simulink model "MotorSlider"  (R2022b)
settings: Solver=VariableStepAuto  StartTime=0.0  StopTime=10  RelTol=1e-3
InitFcn:
  | init_slider
StopFcn:
  | plot_slider_pos
libraries: fl_lib x13, nesl_utility x6, simulink x2, ee_lib x1
settings Model: Creator=lin-t  LastModifiedBy=ddem325
settings DebuggingCC: UnconnectedInputMsg=warning  UnconnectedOutputMsg=warning  UnconnectedLineMsg=warning
settings ModelReferenceCC: EnableRefExpFcnMdlSchedulingChecks=on
settings RTWCC: DLArmComputeVersion=19.05

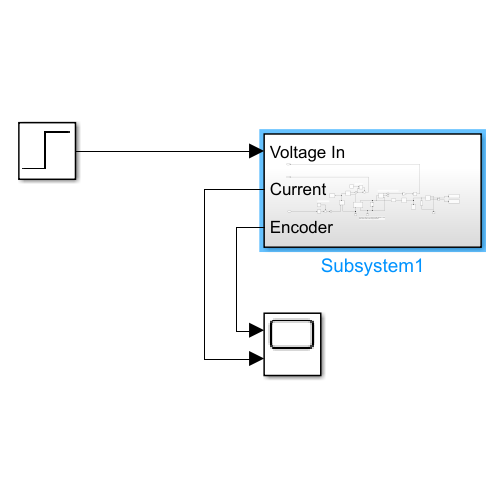
[thumbnail: Simulink's stored preview of the top-level diagram]
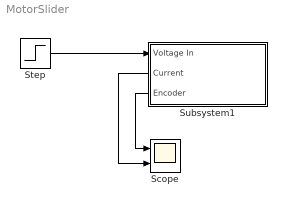
== system MotorSlider ==
  Scope : Scope  NumInputPorts=2
  Step : Step  SampleTime=0
  Subsystem1 : Subsystem
      settings: PortSchema="{\"entries\":[{\"content\":{\"sides\":[{\"content\":{\"connectorIds\":[\"In1\",\"Out1\",\"Out2\"]},\"type\":\"ConnectorPlacement.EquallySpacedRectSide\",\"uuid\":\"37b6e8a3-fab1-42a2-a82e-05d59ddeab9c\"},{\"content\":{\"connectorIds\":[],\"side\":\"RIGHT\"},\"type\":\"ConnectorPlacement.EquallySpacedRectSide\",\"uuid\":\"1ba3cb90-8de0-445d-86e1-8f55e0434744\"},{\"content\":{\"connectorIds\":[],\"side\":\"TOP\"},\"type\":\"ConnectorPlacement.EquallySpacedRectSide\",\"uuid\":\"a1626594-3f4c-461f-b31a-4794292535e7\"}]},\"type\":\"ConnectorPlacement.EquallySpacedConnector\",\"uuid\":\"a2f806fd-1b7f-4e1d-b761-307198229793\"}],\"packageUris\":[\"http://schema.mathworks.com/mf0/Connector/R2020b\"],\"version\":\"1.0\"}"
  wires:
  Subsystem1/2(Encoder) -> Scope/1
  Subsystem1/1(Current) -> Scope/2
  Step/1 -> Subsystem1/1(Voltage In)

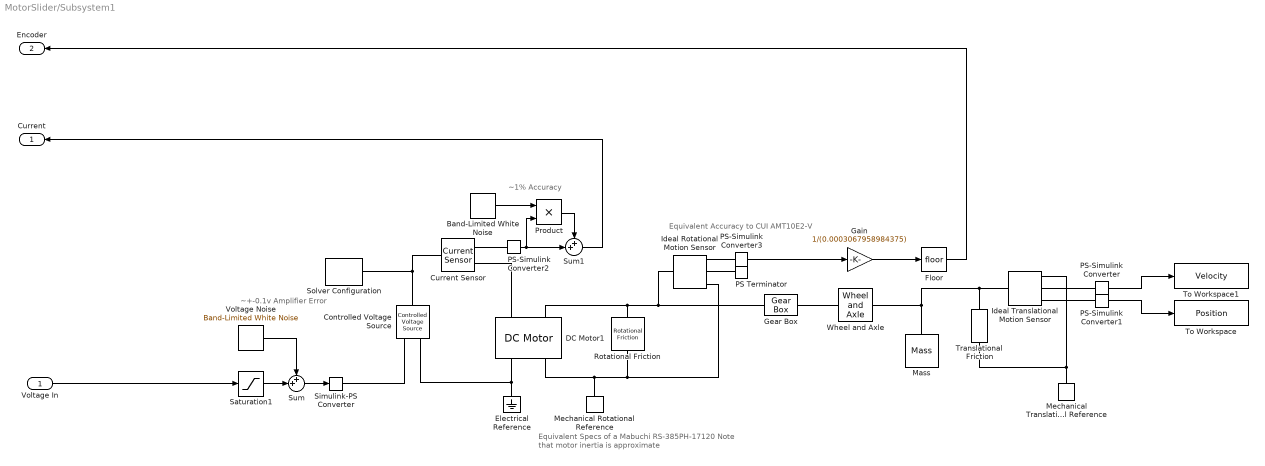
== system MotorSlider/Subsystem1 ==
  note: Equivalent Specs of a Mabuchi RS-385PH-17120
      | Note that motor inertia is approximate
  note: ~1% Accuracy
  note: Equivalent Accuracy to CUI AMT10E2-V
  note: ~+-0.1v Amplifier Error
  Voltage In : Inport
  Band-Limited White Noise : simulink/Sources/Band-Limited White Noise  Cov=[0.0000002]  Ts=0.01  seed=[rand() * 65535]
  Controlled Voltage Source : fl_lib/Electrical/Electrical Sources/Controlled Voltage Source
  Current Sensor : fl_lib/Electrical/Electrical Sensors/Current Sensor
  DC Motor1 : ee_lib/Electromechanical/Brushed Motors/DC Motor  field_option=ee.enum.field_option.pm  Rf=100 Ohm  Lf=1 H  Laf=0.15 H  If0=0 A  parameterization=ee.enum.dcparam_option.circuit_param  Ra=7.71 Ohm  La=12e-6 H  emf_or_torque=ee.enum.emf_or_torque.kv  Kv=0.0251 V/(rad/s)  Ki=6.876e-4 N*m/A  T_stall=0.24e-3 N*m  w_max=19100 rpm  w_rated=15000 rpm  P_rated=0.08 W  V_rated=1.5 V  lam_param=ee.enum.lam_param.damping  i_noload=0 A  V_i_noload=1.5 V  J=1.5e-6 kg*m^2  lam=0 N*m/(rad/s)  speed0=0 rpm  enable_fault_armature=simscape.enum.onoff.off  rev_faulted=1 / 3  G_faulted_armature=1e-5 S  fault_trigger_armature=ee.enum.faults.faultTrigger.temporal  t_fault_armature=1 s  max_permissible_current_armature=inf A  t_fail_on_current_armature=1 s  enable_fault_field=simscape.enum.onoff.off  G_faulted_field=1e-5 S  fault_trigger_field=ee.enum.faults.faultTrigger.temporal  t_fault_field=1 s  max_permissible_current_field=inf A  t_fail_on_current_field=1 s  fault_action=simscape.enum.assert.action.none  alpha=3.93e-3 1/K  Tmeas=25 degC  thermal_mass=100 J/K  initial_temperature=25 degC
  Electrical Reference : fl_lib/Electrical/Electrical Elements/Electrical Reference
  Floor : Rounding
  Gain : Gain  Gain=1/(0.0003067958984375)
  Gear Box : fl_lib/Mechanical/Mechanisms/Gear Box  ratio=3  t_in_specify=off  t_in_priority=None  t_in=0 N*m  t_in_nominal_specify=off  t_in_nominal_unit=N*m  t_in_nominal_value=1  t_out_specify=off  t_out_priority=None  t_out=0 N*m  t_out_nominal_specify=off  t_out_nominal_unit=N*m  t_out_nominal_value=1
  Ideal Rotational Motion Sensor : fl_lib/Mechanical/Mechanical Sensors/Ideal Rotational Motion Sensor  reference=foundation.enum.MeasurementReference.difference  acceleration_port=false  velocity_port=true  position_port=true  wrap_angle=simscape.enum.onoff.off  offset=0 rad
  Ideal Translational Motion Sensor : fl_lib/Mechanical/Mechanical Sensors/Ideal Translational Motion Sensor  reference=foundation.enum.MeasurementReference.difference  acceleration_port=false  velocity_port=true  position_port=true  offset=0 m
  Mass : fl_lib/Mechanical/Translational Elements/Mass  mass=1.5 kg  num_ports=foundation.enum.numPorts2.one  v_specify=off  v_priority=High  v=0 m/s  v_nominal_specify=off  v_nominal_unit=m/s  v_nominal_value=1  f_specify=off  f_priority=None  f=0 N  f_nominal_specify=off  f_nominal_unit=N  f_nominal_value=1
  Mechanical Rotational Reference : fl_lib/Mechanical/Rotational Elements/Mechanical Rotational Reference
  Mechanical Translational Reference : fl_lib/Mechanical/Translational Elements/Mechanical Translational Reference
  PS Terminator : fl_lib/Physical Signals/Sinks/PS Terminator
  PS-Simulink Converter{,1..3} (4 alike) : nesl_utility/PS-Simulink Converter  PhysicalDomain=network_engine_domain  SubClassName=ps_output  LeftPortType=input  RightPortType=output  PseudoPeriodic=off  Frequencies=[]  VectorFormat=1-D array  Unit=inherit  AffineConversion=off
  Product : Product
  Rotational Friction : fl_lib/Mechanical/Rotational Elements/Rotational Friction  brkwy_trq=1e-5 N*m  brkwy_vel=1e-9 rad/s  Col_trq=1e-9 N*m  visc_coef=2.148e-6 N*m/(rad/s)  w_specify=off  w_priority=None  w=0 rad/s  w_nominal_specify=off  w_nominal_unit=rad/s  w_nominal_value=1  t_specify=off  t_priority=None  t=0 N*m  t_nominal_specify=off  t_nominal_unit=N*m  t_nominal_value=1
  Saturation1 : Saturate  UpperLimit=15  LowerLimit=-15
  Simulink-PS Converter : nesl_utility/Simulink-PS Converter  PhysicalDomain=network_engine_domain  SubClassName=ps_input  LeftPortType=input  RightPortType=output  PseudoPeriodic=off  Frequencies=[]  NoiseDistribution=none  NoiseParameters=[]  Unit=1  AffineConversion=off  FilteringAndDerivatives=provide  SimscapeFilterOrder=1  InputFilterTimeConstant=0.001  UdotUserProvided=0
  Solver Configuration : nesl_utility/Solver Configuration  PhysicalDomain=network_engine_domain  SubClassName=solver  LeftPortType=input  RightPortType=generic  Tones=[]  Harmonics=[]  SimulateNoise=off  Profile=off  UseLocalSampling=off  EnableSwitchedLinearOptims=on  FrequencyDomain=off  UseCCode=off  RelTol=0.001  AbsTol=1e-06  MinStep=1e-09  ToWorkspace=off  RevertToSquareIcSolve=off  NumHomotopyIterations=100  PhasorMode=off  PhasorModeNumHarmonics=1  ConsistencySolver=NEWTON_FTOL  IndexReductionMethod=DerivativeReplacement  DoDC=off  ResidualTolerance=1e-09  ConsistencyTolSource=GLOBAL  ConsistencyAbsTol=0.001  ConsistencyRelTol=0.001  ConsistencyTolFactor=0.001  UseLocalSolver=off  LocalSolverChoice=NE_BACKWARD_EULER_ADVANCER  ResolveIndetEquations=on  FunctionEvalNumThread=1  LocalSolverSampleTime=0.001  DoFixedCost=off  MaxNonlinIter=3  MaxModeIter=2  ComputeImpulses=off  ImpulseIterations=2  LinearAlgebra=auto  LinearAlgebraNumThread=0  EquationFormulation=NE_TIME_EF  DelaysMemoryBudget=1024  AutomaticFiltering=on  FilteringTimeConstant=0.001  PartitionStorageMethod=AS_NEEDED  PartitionMemoryBudget=1024  PartitionMethod=ROBUST
  Sum : Sum  Inputs=++|
  Sum1 : Sum  Inputs=++|
  To Workspace : ToWorkspace  VariableName=Position  SaveFormat=Timeseries  SampleTime=-1
  To Workspace1 : ToWorkspace  VariableName=Velocity  SaveFormat=Timeseries  SampleTime=-1
  Translational Friction : fl_lib/Mechanical/Translational Elements/Translational Friction  brkwy_frc=0.2 N  brkwy_vel=0.01 m/s  Col_frc=0.05 N  visc_coef=0.05 N/(m/s)  v_specify=off  v_priority=None  v=0 m/s  v_nominal_specify=off  v_nominal_unit=m/s  v_nominal_value=1  f_specify=off  f_priority=None  f=0 N  f_nominal_specify=off  f_nominal_unit=N  f_nominal_value=1
      settings: InternalSimscapePortConfiguration="{\"Bottom\":[],\"Left\":[{\"id\":\"R\",\"label\":\"R\",\"type\":\"foundation.mechanical.translational.translational\"}],\"Right\":[{\"id\":\"C\",\"label\":\"C\",\"type\":\"foundation.mechanical.translational.translational\"}],\"Top\":[]}"
  Voltage Noise : simulink/Sources/Band-Limited White Noise  Cov=[0.00001]  Ts=0.01  seed=[rand() * 65535]
  Wheel and Axle : fl_lib/Mechanical/Mechanisms/Wheel and Axle  R=0.5 cm  or=1  t_specify=off  t_priority=None  t=0 N*m  t_nominal_specify=off  t_nominal_unit=N*m  t_nominal_value=1  f_specify=off  f_priority=None  f=0 N  f_nominal_specify=off  f_nominal_unit=N  f_nominal_value=1
  Current : Outport
  Encoder : Outport  Port=2
  wires:
  Sum1/1 -> Current/1
  PS-Simulink Converter2/1 -> Product/2, Sum1/2
  Saturation1/1 -> Sum/2
  Sum/1 -> Simulink-PS Converter/1
  Voltage In/1 -> Saturation1/1
  PS-Simulink Converter3/1 -> Gain/1
  Gain/1 -> Floor/1
  Band-Limited White Noise/1 -> Product/1
  Floor/1 -> Encoder/1
  Product/1 -> Sum1/1
  Voltage Noise/1 -> Sum/1
  PS-Simulink Converter1/1 -> To Workspace/1
  PS-Simulink Converter/1 -> To Workspace1/1
  connections:
  Electrical Reference/LConn1 -- Controlled Voltage Source/RConn2 -- DC Motor1/RConn1
  Wheel and Axle/RConn1 -- Translational Friction/LConn1 -- Ideal Translational Motion Sensor/LConn1 -- Mass/LConn1
  Ideal Translational Motion Sensor/RConn3 -- PS-Simulink Converter1/LConn1
  DC Motor1/RConn2 -- Ideal Rotational Motion Sensor/RConn1 -- Rotational Friction/RConn1 -- Mechanical Rotational Reference/LConn1
  PS Terminator/LConn1 -- Ideal Rotational Motion Sensor/RConn2
  PS-Simulink Converter3/LConn1 -- Ideal Rotational Motion Sensor/RConn3
  Controlled Voltage Source/LConn1 -- Solver Configuration/RConn1 -- Current Sensor/LConn1
  Ideal Rotational Motion Sensor/LConn1 -- Rotational Friction/LConn1 -- DC Motor1/LConn2 -- Gear Box/LConn1
  Ideal Translational Motion Sensor/RConn2 -- PS-Simulink Converter/LConn1
  Mechanical Translational Reference/LConn1 -- Translational Friction/RConn1 -- Ideal Translational Motion Sensor/RConn1
  Simulink-PS Converter/RConn1 -- Controlled Voltage Source/RConn1
  Current Sensor/RConn2 -- DC Motor1/LConn1
  PS-Simulink Converter2/LConn1 -- Current Sensor/RConn1
  Gear Box/RConn1 -- Wheel and Axle/LConn1
